simulink model "RapiroArduino"  (R2014a)
settings: Solver=ode3  SolverMode=SingleTasking  StartTime=0.0  StopTime=30  RelTol=1e-3
InitFcn:
  | Ts = 1e-6
libraries: arduinolib x6, simulink x5
settings Model: ExtModeTrigDuration=2  Creator=akaushik  LastModifiedBy=yanlianz
settings OptimizationCC: OptimizeModelRefInitCode=on  LifeSpan=1
settings DebuggingCC: UnderspecifiedInitializationDetection=Classic  SolverPrmCheckMsg=none
settings HardwareCC: ProdBitPerInt=16  ProdBitPerPointer=8  ProdIntDivRoundTo=Zero  ProdEndianess=LittleEndian  ProdWordSize=8  ProdHWDeviceType=Atmel->AVR
settings RTWCC: SystemTargetFile=realtime.tlc  GenerateMakefile=off  TemplateMakefile=realtime.tmf  Description=Run on Target Hardware  RTWVerbose=off  ProcessScript=realtime_make_rtw_hook
settings STFCustomTargetCC: TargetLibSuffix=.a  GenerateSampleERTMain=on  ConcurrentExecutionCompliant=off  GeneratePreprocessorConditionals=Use local settings  ERTCustomFileBanners=on  SupportNonInlinedSFcns=off  SupportVariableSizeSignals=on  MATLABClassNameForMDSCustomization=Simulink.SoftwareTarget.ERTCustomization  GRTInterface=off  SystemTargetFile=realtime.tlc
settings ERTTargetCC: CombineOutputUpdateFcns=off  SupportContinuousTime=on  SupportVariableSizeSignals=on  ExtModeTransport=3  ExtModeMexFile=ext_serial_win32_comm  ExtModeMexArgs=0 1 9600  ERTSrcFileBannerTemplate=realtime_code_template.cgt  ERTHdrFileBannerTemplate=realtime_code_template.cgt  ERTDataSrcFileTemplate=realtime_code_template.cgt  ERTDataHdrFileTemplate=realtime_code_template.cgt  ERTCustomFileTemplate=realtime_file_process.tlc

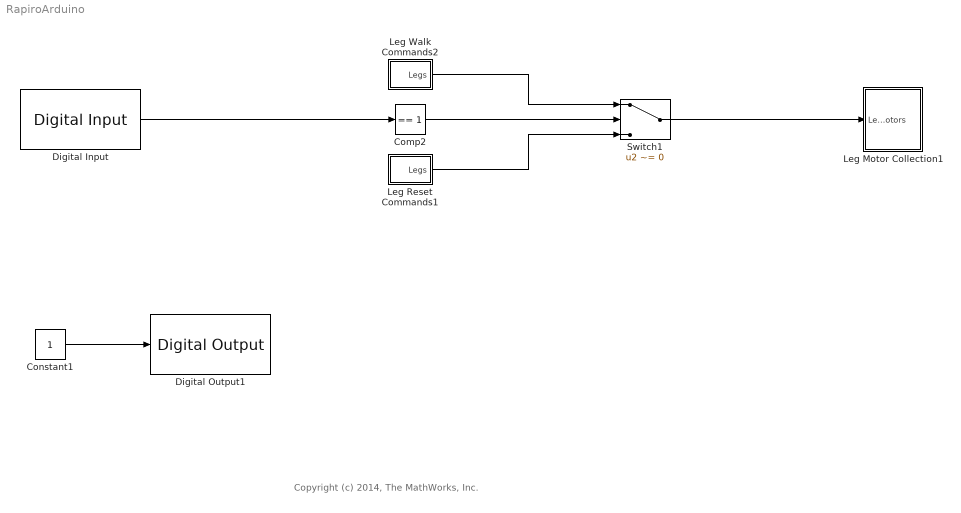
== system RapiroArduino ==
  note: Copyright (c) 2014, The MathWorks, Inc.
  Comp2 : simulink/Logic and Bit Operations/Compare To Constant  relop===  const=1  OutDataTypeStr=boolean
  Constant1 : Constant
  Digital Input : arduinolib/Digital Input  pinNumber=3  sampleTime=1e-2
  Digital Output1 : arduinolib/Digital Output  pinNumber=A3
  Leg Motor Collection1 : Subsystem
  Leg Reset Commands1 : Subsystem
  Leg Walk Commands2 : Subsystem
  Switch1 : Switch  Criteria=u2 ~= 0  OutDataTypeStr=uint8
  wires:
  Switch1/1 -> Leg Motor Collection1/1(Leg_Motors)
  Constant1/1 -> Digital Output1/1
  Leg Walk Commands2/1(Legs) -> Switch1/1
  Leg Reset Commands1/1(Legs) -> Switch1/3
  Comp2/1 -> Switch1/2
  Digital Input/1 -> Comp2/1

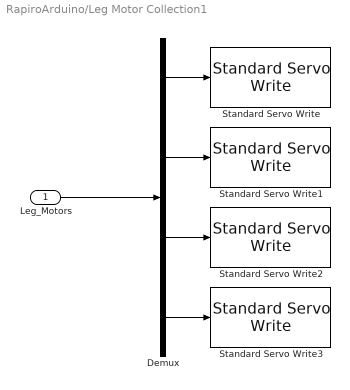
== system RapiroArduino/Leg Motor Collection1 ==
  Leg_Motors : Inport
  Demux : Demux
  Standard Servo Write : arduinolib/Standard Servo Write  pinNumber=4
  Standard Servo Write1 : arduinolib/Standard Servo Write  pinNumber=2
  Standard Servo Write2 : arduinolib/Standard Servo Write  pinNumber=A1
  Standard Servo Write3 : arduinolib/Standard Servo Write  pinNumber=A2
  wires:
  Leg_Motors/1 -> Demux/1
  Demux/1 -> Standard Servo Write/1
  Demux/4 -> Standard Servo Write3/1
  Demux/2 -> Standard Servo Write1/1
  Demux/3 -> Standard Servo Write2/1

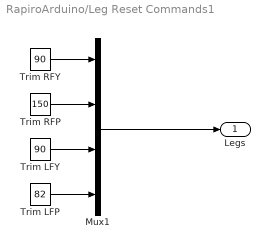
== system RapiroArduino/Leg Reset Commands1 ==
  Mux1 : Mux
  Trim LFP : Constant  Value=82  OutDataTypeStr=uint8
  Trim LFY : Constant  Value=90  OutDataTypeStr=uint8
  Trim RFP : Constant  Value=150  OutDataTypeStr=uint8
  Trim RFY : Constant  Value=90  OutDataTypeStr=uint8
  Legs : Outport
  wires:
  Trim LFY/1 -> Mux1/3
  Trim LFP/1 -> Mux1/4
  Trim RFY/1 -> Mux1/1
  Trim RFP/1 -> Mux1/2
  Mux1/1 -> Legs/1

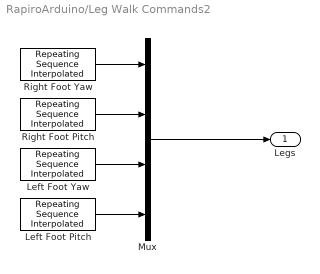
== system RapiroArduino/Leg Walk Commands2 ==
  Left Foot Pitch : simulink/Sources/Repeating Sequence Interpolated  OutValues=[120 90 80 70 90 110 120]  TimeValues=[0 1 2 3 4 5 6]*0.001  LookUpMeth=Interpolation-Use End Values  tsamp=Ts  OutMin=[]  OutMax=[]  OutDataTypeStr=uint8  OutputDataTypeScalingMode=uint8  OutDataType=fixdt(0,8)  OutScaling=2^-10
  Left Foot Yaw : simulink/Sources/Repeating Sequence Interpolated  OutValues=[80 70 70 100 110 110 80]  TimeValues=[0 1 2 3 4 5 6]*0.001  LookUpMeth=Interpolation-Use End Values  tsamp=Ts  OutMin=[]  OutMax=[]  OutDataTypeStr=uint8  OutputDataTypeScalingMode=uint8  OutDataType=fixdt(0,8)  OutScaling=2^-10
  Mux : Mux
  Right Foot Pitch : simulink/Sources/Repeating Sequence Interpolated  OutValues=[180 160 150 140 150 160 180]  TimeValues=[0 1 2 3 4 5 6]*0.001  LookUpMeth=Interpolation-Use End Values  tsamp=Ts  OutMin=[]  OutMax=[]  OutDataTypeStr=uint8  OutputDataTypeScalingMode=uint8  OutDataType=fixdt(0,8)  OutScaling=2^-10
  Right Foot Yaw : simulink/Sources/Repeating Sequence Interpolated  OutValues=[80 70 70 100 110 110 80]  TimeValues=[0 1 2 3 4 5 6]*0.001  LookUpMeth=Interpolation-Use End Values  tsamp=Ts  OutMin=[]  OutMax=[]  OutDataTypeStr=uint8  OutputDataTypeScalingMode=uint8  OutDataType=fixdt(0,8)  OutScaling=2^-10
  Legs : Outport
  wires:
  Left Foot Pitch/1 -> Mux/4
  Left Foot Yaw/1 -> Mux/3
  Right Foot Yaw/1 -> Mux/1
  Right Foot Pitch/1 -> Mux/2
  Mux/1 -> Legs/1
